simulink model "pi_choiceIface"  (R2018b)
settings: Solver=FixedStepDiscrete  StartTime=0.0  StopTime=10.0  RelTol=1e-3
undefined symbols (not defined in the file): boolAliasMember, boolMember, choiceAliasesMember, choiceBuiltInMember, choiceIdx, choiceOfFixedSizeSeqOfsMember, choiceOfVarSizeSeqOfsMember, enumAliasMember, enumMember, ia5StringFixedSizeAliasMember, ia5StringFixedSizeMember, ia5StringVarSizeAliasMember, ia5StringVarSizeMember, integerAliasMember, integerMember, octetStringFixedSizeAliasMember, octetStringFixedSizeMember, octetStringVarSizeAliasMember, octetStringVarSizeMember, realAliasMember, realMember, seqAliasesMember, seqBuiltInMember, seqOfFixedSizeSeqOfsMember, seqOfVarSizeSeqOfsMember
settings Model: Creator=matlab  LastModifiedBy=matlab
settings DataIOCC: SaveOutput=off  SignalLogging=off  SaveTime=off
settings OptimizationCC: DefaultParameterBehavior=Inlined  EnhancedBackFolding=on  PassReuseOutputArgsAs=Individual arguments  OptimizeBlockOrder=speed  DifferentSizesBufferReuse=on  OptimizationCustomize=off
settings DebuggingCC: ParameterTunabilityLossMsg=error
settings SFSimCC: MATLABDynamicMemAlloc=off
settings RTWCC: SystemTargetFile=ert.tlc  TemplateMakefile=ert_default_tmf  PostCodeGenCommand=packNGo(buildInfo);  GenerateReport=on  IncludeHyperlinkInReport=on  LaunchReport=on  GenerateTraceInfo=on  GenerateTraceReport=on  GenerateTraceReportSl=on  GenerateTraceReportSf=on  GenerateTraceReportEml=on
settings CodeAppCC: ForceParamTrailComments=on  IgnoreCustomStorageClasses=off  OperatorAnnotations=on  SimulinkDataObjDesc=on  SFDataObjDesc=on  InsertBlockDesc=on
settings ERTTargetCC: TargetLangStandard=C99 (ISO)  GenerateSampleERTMain=on  InlinedParameterPlacement=NonHierarchical  ERTCustomFileTemplate=example_file_process.tlc

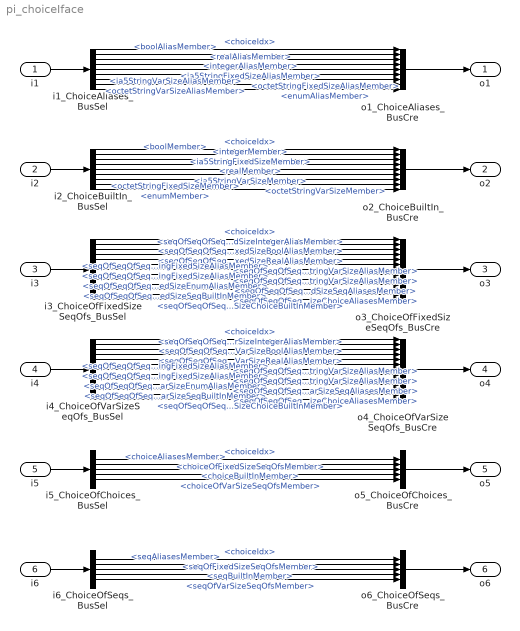
== system pi_choiceIface ==
  i1 : Inport  OutDataTypeStr=Bus: ChoiceAliases  BusOutputAsStruct=on
  i2 : Inport  Port=2  OutDataTypeStr=Bus: ChoiceBuiltIn  BusOutputAsStruct=on
  i3 : Inport  Port=3  OutDataTypeStr=Bus: ChoiceOfFixedSizeSeqOfs  BusOutputAsStruct=on
  i4 : Inport  Port=4  OutDataTypeStr=Bus: ChoiceOfVarSizeSeqOfs  BusOutputAsStruct=on
  i5 : Inport  Port=5  OutDataTypeStr=Bus: ChoiceOfChoices  BusOutputAsStruct=on
  i6 : Inport  Port=6  OutDataTypeStr=Bus: ChoiceOfSeqs  BusOutputAsStruct=on
  i1_ChoiceAliases_BusSel : BusSelector  OutputSignals=choiceIdx,boolAliasMember,integerAliasMember,realAliasMember,ia5StringFixedSizeAliasMember,ia5StringVarSizeAliasMember,octetStringFixedSizeAliasMember,octetStringVarSizeAliasMember,enumAliasMember
  i2_ChoiceBuiltIn_BusSel : BusSelector  OutputSignals=choiceIdx,boolMember,integerMember,realMember,ia5StringFixedSizeMember,ia5StringVarSizeMember,octetStringFixedSizeMember,octetStringVarSizeMember,enumMember
  i3_ChoiceOfFixedSizeSeqOfs_BusSel : BusSelector  OutputSignals=choiceIdx,seqOfSeqOfSeqOfFixedSizeBoolAliasMember,seqOfSeqOfSeqOfFixedSizeIntegerAliasMember,seqOfSeqOfSeqOfFixedSizeRealAliasMember,seqOfSeqOfSeqOfFixedSizeIA5StringFixedSizeAliasMember,seqOfSeqOfSeqOfFixedSizeIA5StringVarSizeAliasMember,seqOfSeqOfSeqOfFixedSizeOctetStringFixedSizeAliasMember,seqOfSeqOfSeqOfFixedSizeOctetStringVarSizeAliasMember,seqOfSeqOfSeqOfFixedSizeEnumAliasMember,seqOfSeqOfSeqOfFixedSizeSeqAliasesMember,seqOfSeqOfSeqOfFixedSizeSeqBuiltInMember,seqOfSeqOfSeqOfFixedSizeChoiceAliasesMember,seqOfSeqOfSeqOfFixedSizeChoiceBuiltInMember
  i4_ChoiceOfVarSizeSeqOfs_BusSel : BusSelector  OutputSignals=choiceIdx,seqOfSeqOfSeqOfVarSizeBoolAliasMember,seqOfSeqOfSeqOfVarSizeIntegerAliasMember,seqOfSeqOfSeqOfVarSizeRealAliasMember,seqOfSeqOfSeqOfVarSizeIA5StringFixedSizeAliasMember,seqOfSeqOfSeqOfVarSizeIA5StringVarSizeAliasMember,seqOfSeqOfSeqOfVarSizeOctetStringFixedSizeAliasMember,seqOfSeqOfSeqOfVarSizeOctetStringVarSizeAliasMember,seqOfSeqOfSeqOfVarSizeEnumAliasMember,seqOfSeqOfSeqOfVarSizeSeqAliasesMember,seqOfSeqOfSeqOfVarSizeSeqBuiltInMember,seqOfSeqOfSeqOfVarSizeChoiceAliasesMember,seqOfSeqOfSeqOfVarSizeChoiceBuiltInMember
  i5_ChoiceOfChoices_BusSel : BusSelector  OutputSignals=choiceIdx,choiceAliasesMember,choiceBuiltInMember,choiceOfFixedSizeSeqOfsMember,choiceOfVarSizeSeqOfsMember
  i6_ChoiceOfSeqs_BusSel : BusSelector  OutputSignals=choiceIdx,seqAliasesMember,seqBuiltInMember,seqOfFixedSizeSeqOfsMember,seqOfVarSizeSeqOfsMember
  o1_ChoiceAliases_BusCre : BusCreator  Inputs=choiceIdx,boolAliasMember,integerAliasMember,realAliasMember,ia5StringFixedSizeAliasMember,ia5StringVarSizeAliasMember,octetStringFixedSizeAliasMember,octetStringVarSizeAliasMember,enumAliasMember  OutDataTypeStr=Bus: ChoiceAliases  NonVirtualBus=on
  o2_ChoiceBuiltIn_BusCre : BusCreator  Inputs=choiceIdx,boolMember,integerMember,realMember,ia5StringFixedSizeMember,ia5StringVarSizeMember,octetStringFixedSizeMember,octetStringVarSizeMember,enumMember  OutDataTypeStr=Bus: ChoiceBuiltIn  NonVirtualBus=on
  o3_ChoiceOfFixedSizeSeqOfs_BusCre : BusCreator  Inputs=choiceIdx,seqOfSeqOfSeqOfFixedSizeBoolAliasMember,seqOfSeqOfSeqOfFixedSizeIntegerAliasMember,seqOfSeqOfSeqOfFixedSizeRealAliasMember,seqOfSeqOfSeqOfFixedSizeIA5StringFixedSizeAliasMember,seqOfSeqOfSeqOfFixedSizeIA5StringVarSizeAliasMember,seqOfSeqOfSeqOfFixedSizeOctetStringFixedSizeAliasMember,seqOfSeqOfSeqOfFixedSizeOctetStringVarSizeAliasMember,seqOfSeqOfSeqOfFixedSizeEnumAliasMember,seqOfSeqOfSeqOfFixedSizeSeqAliasesMember,seqOfSeqOfSeqOfFixedSizeSeqBuiltInMember,seqOfSeqOfSeqOfFixedSizeChoiceAliasesMember,seqOfSeqOfSeqOfFixedSizeChoiceBuiltInMember  OutDataTypeStr=Bus: ChoiceOfFixedSizeSeqOfs  NonVirtualBus=on
  o4_ChoiceOfVarSizeSeqOfs_BusCre : BusCreator  Inputs=choiceIdx,seqOfSeqOfSeqOfVarSizeBoolAliasMember,seqOfSeqOfSeqOfVarSizeIntegerAliasMember,seqOfSeqOfSeqOfVarSizeRealAliasMember,seqOfSeqOfSeqOfVarSizeIA5StringFixedSizeAliasMember,seqOfSeqOfSeqOfVarSizeIA5StringVarSizeAliasMember,seqOfSeqOfSeqOfVarSizeOctetStringFixedSizeAliasMember,seqOfSeqOfSeqOfVarSizeOctetStringVarSizeAliasMember,seqOfSeqOfSeqOfVarSizeEnumAliasMember,seqOfSeqOfSeqOfVarSizeSeqAliasesMember,seqOfSeqOfSeqOfVarSizeSeqBuiltInMember,seqOfSeqOfSeqOfVarSizeChoiceAliasesMember,seqOfSeqOfSeqOfVarSizeChoiceBuiltInMember  OutDataTypeStr=Bus: ChoiceOfVarSizeSeqOfs  NonVirtualBus=on
  o5_ChoiceOfChoices_BusCre : BusCreator  Inputs=choiceIdx,choiceAliasesMember,choiceBuiltInMember,choiceOfFixedSizeSeqOfsMember,choiceOfVarSizeSeqOfsMember  OutDataTypeStr=Bus: ChoiceOfChoices  NonVirtualBus=on
  o6_ChoiceOfSeqs_BusCre : BusCreator  Inputs=choiceIdx,seqAliasesMember,seqBuiltInMember,seqOfFixedSizeSeqOfsMember,seqOfVarSizeSeqOfsMember  OutDataTypeStr=Bus: ChoiceOfSeqs  NonVirtualBus=on
  o1 : Outport  OutDataTypeStr=Bus: ChoiceAliases  BusOutputAsStruct=on
  o2 : Outport  Port=2  OutDataTypeStr=Bus: ChoiceBuiltIn  BusOutputAsStruct=on
  o3 : Outport  Port=3  OutDataTypeStr=Bus: ChoiceOfFixedSizeSeqOfs  BusOutputAsStruct=on
  o4 : Outport  Port=4  OutDataTypeStr=Bus: ChoiceOfVarSizeSeqOfs  BusOutputAsStruct=on
  o5 : Outport  Port=5  OutDataTypeStr=Bus: ChoiceOfChoices  BusOutputAsStruct=on
  o6 : Outport  Port=6  OutDataTypeStr=Bus: ChoiceOfSeqs  BusOutputAsStruct=on
  wires:
  i1/1 -> i1_ChoiceAliases_BusSel/1
  i2/1 -> i2_ChoiceBuiltIn_BusSel/1
  i3/1 -> i3_ChoiceOfFixedSizeSeqOfs_BusSel/1
  i4/1 -> i4_ChoiceOfVarSizeSeqOfs_BusSel/1
  i5/1 -> i5_ChoiceOfChoices_BusSel/1
  i6/1 -> i6_ChoiceOfSeqs_BusSel/1
  o1_ChoiceAliases_BusCre/1 -> o1/1
  o2_ChoiceBuiltIn_BusCre/1 -> o2/1
  o3_ChoiceOfFixedSizeSeqOfs_BusCre/1 -> o3/1
  o4_ChoiceOfVarSizeSeqOfs_BusCre/1 -> o4/1
  o5_ChoiceOfChoices_BusCre/1 -> o5/1
  o6_ChoiceOfSeqs_BusCre/1 -> o6/1
  i1_ChoiceAliases_BusSel/1 -> o1_ChoiceAliases_BusCre/1  "<choiceIdx>"
  i1_ChoiceAliases_BusSel/2 -> o1_ChoiceAliases_BusCre/2  "<boolAliasMember>"
  i1_ChoiceAliases_BusSel/3 -> o1_ChoiceAliases_BusCre/3  "<integerAliasMember>"
  i1_ChoiceAliases_BusSel/4 -> o1_ChoiceAliases_BusCre/4  "<realAliasMember>"
  i1_ChoiceAliases_BusSel/5 -> o1_ChoiceAliases_BusCre/5  "<ia5StringFixedSizeAliasMember>"
  i1_ChoiceAliases_BusSel/6 -> o1_ChoiceAliases_BusCre/6  "<ia5StringVarSizeAliasMember>"
  i1_ChoiceAliases_BusSel/7 -> o1_ChoiceAliases_BusCre/7  "<octetStringFixedSizeAliasMember>"
  i1_ChoiceAliases_BusSel/8 -> o1_ChoiceAliases_BusCre/8  "<octetStringVarSizeAliasMember>"
  i1_ChoiceAliases_BusSel/9 -> o1_ChoiceAliases_BusCre/9  "<enumAliasMember>"
  i2_ChoiceBuiltIn_BusSel/1 -> o2_ChoiceBuiltIn_BusCre/1  "<choiceIdx>"
  i2_ChoiceBuiltIn_BusSel/2 -> o2_ChoiceBuiltIn_BusCre/2  "<boolMember>"
  i2_ChoiceBuiltIn_BusSel/3 -> o2_ChoiceBuiltIn_BusCre/3  "<integerMember>"
  i2_ChoiceBuiltIn_BusSel/4 -> o2_ChoiceBuiltIn_BusCre/4  "<realMember>"
  i2_ChoiceBuiltIn_BusSel/5 -> o2_ChoiceBuiltIn_BusCre/5  "<ia5StringFixedSizeMember>"
  i2_ChoiceBuiltIn_BusSel/6 -> o2_ChoiceBuiltIn_BusCre/6  "<ia5StringVarSizeMember>"
  i2_ChoiceBuiltIn_BusSel/7 -> o2_ChoiceBuiltIn_BusCre/7  "<octetStringFixedSizeMember>"
  i2_ChoiceBuiltIn_BusSel/8 -> o2_ChoiceBuiltIn_BusCre/8  "<octetStringVarSizeMember>"
  i2_ChoiceBuiltIn_BusSel/9 -> o2_ChoiceBuiltIn_BusCre/9  "<enumMember>"
  i3_ChoiceOfFixedSizeSeqOfs_BusSel/1 -> o3_ChoiceOfFixedSizeSeqOfs_BusCre/1  "<choiceIdx>"
  i3_ChoiceOfFixedSizeSeqOfs_BusSel/2 -> o3_ChoiceOfFixedSizeSeqOfs_BusCre/2  "<seqOfSeqOfSeqOfFixedSizeBoolAliasMember>"
  i3_ChoiceOfFixedSizeSeqOfs_BusSel/3 -> o3_ChoiceOfFixedSizeSeqOfs_BusCre/3  "<seqOfSeqOfSeqOfFixedSizeIntegerAliasMember>"
  i3_ChoiceOfFixedSizeSeqOfs_BusSel/4 -> o3_ChoiceOfFixedSizeSeqOfs_BusCre/4  "<seqOfSeqOfSeqOfFixedSizeRealAliasMember>"
  i3_ChoiceOfFixedSizeSeqOfs_BusSel/5 -> o3_ChoiceOfFixedSizeSeqOfs_BusCre/5  "<seqOfSeqOfSeqOfFixedSizeIA5StringFixedSizeAliasMember>"
  i3_ChoiceOfFixedSizeSeqOfs_BusSel/6 -> o3_ChoiceOfFixedSizeSeqOfs_BusCre/6  "<seqOfSeqOfSeqOfFixedSizeIA5StringVarSizeAliasMember>"
  i3_ChoiceOfFixedSizeSeqOfs_BusSel/7 -> o3_ChoiceOfFixedSizeSeqOfs_BusCre/7  "<seqOfSeqOfSeqOfFixedSizeOctetStringFixedSizeAliasMember>"
  i3_ChoiceOfFixedSizeSeqOfs_BusSel/8 -> o3_ChoiceOfFixedSizeSeqOfs_BusCre/8  "<seqOfSeqOfSeqOfFixedSizeOctetStringVarSizeAliasMember>"
  i3_ChoiceOfFixedSizeSeqOfs_BusSel/9 -> o3_ChoiceOfFixedSizeSeqOfs_BusCre/9  "<seqOfSeqOfSeqOfFixedSizeEnumAliasMember>"
  i3_ChoiceOfFixedSizeSeqOfs_BusSel/10 -> o3_ChoiceOfFixedSizeSeqOfs_BusCre/10  "<seqOfSeqOfSeqOfFixedSizeSeqAliasesMember>"
  i3_ChoiceOfFixedSizeSeqOfs_BusSel/11 -> o3_ChoiceOfFixedSizeSeqOfs_BusCre/11  "<seqOfSeqOfSeqOfFixedSizeSeqBuiltInMember>"
  i3_ChoiceOfFixedSizeSeqOfs_BusSel/12 -> o3_ChoiceOfFixedSizeSeqOfs_BusCre/12  "<seqOfSeqOfSeqOfFixedSizeChoiceAliasesMember>"
  i3_ChoiceOfFixedSizeSeqOfs_BusSel/13 -> o3_ChoiceOfFixedSizeSeqOfs_BusCre/13  "<seqOfSeqOfSeqOfFixedSizeChoiceBuiltInMember>"
  i4_ChoiceOfVarSizeSeqOfs_BusSel/1 -> o4_ChoiceOfVarSizeSeqOfs_BusCre/1  "<choiceIdx>"
  i4_ChoiceOfVarSizeSeqOfs_BusSel/2 -> o4_ChoiceOfVarSizeSeqOfs_BusCre/2  "<seqOfSeqOfSeqOfVarSizeBoolAliasMember>"
  i4_ChoiceOfVarSizeSeqOfs_BusSel/3 -> o4_ChoiceOfVarSizeSeqOfs_BusCre/3  "<seqOfSeqOfSeqOfVarSizeIntegerAliasMember>"
  i4_ChoiceOfVarSizeSeqOfs_BusSel/4 -> o4_ChoiceOfVarSizeSeqOfs_BusCre/4  "<seqOfSeqOfSeqOfVarSizeRealAliasMember>"
  i4_ChoiceOfVarSizeSeqOfs_BusSel/5 -> o4_ChoiceOfVarSizeSeqOfs_BusCre/5  "<seqOfSeqOfSeqOfVarSizeIA5StringFixedSizeAliasMember>"
  i4_ChoiceOfVarSizeSeqOfs_BusSel/6 -> o4_ChoiceOfVarSizeSeqOfs_BusCre/6  "<seqOfSeqOfSeqOfVarSizeIA5StringVarSizeAliasMember>"
  i4_ChoiceOfVarSizeSeqOfs_BusSel/7 -> o4_ChoiceOfVarSizeSeqOfs_BusCre/7  "<seqOfSeqOfSeqOfVarSizeOctetStringFixedSizeAliasMember>"
  i4_ChoiceOfVarSizeSeqOfs_BusSel/8 -> o4_ChoiceOfVarSizeSeqOfs_BusCre/8  "<seqOfSeqOfSeqOfVarSizeOctetStringVarSizeAliasMember>"
  i4_ChoiceOfVarSizeSeqOfs_BusSel/9 -> o4_ChoiceOfVarSizeSeqOfs_BusCre/9  "<seqOfSeqOfSeqOfVarSizeEnumAliasMember>"
  i4_ChoiceOfVarSizeSeqOfs_BusSel/10 -> o4_ChoiceOfVarSizeSeqOfs_BusCre/10  "<seqOfSeqOfSeqOfVarSizeSeqAliasesMember>"
  i4_ChoiceOfVarSizeSeqOfs_BusSel/11 -> o4_ChoiceOfVarSizeSeqOfs_BusCre/11  "<seqOfSeqOfSeqOfVarSizeSeqBuiltInMember>"
  i4_ChoiceOfVarSizeSeqOfs_BusSel/12 -> o4_ChoiceOfVarSizeSeqOfs_BusCre/12  "<seqOfSeqOfSeqOfVarSizeChoiceAliasesMember>"
  i4_ChoiceOfVarSizeSeqOfs_BusSel/13 -> o4_ChoiceOfVarSizeSeqOfs_BusCre/13  "<seqOfSeqOfSeqOfVarSizeChoiceBuiltInMember>"
  i5_ChoiceOfChoices_BusSel/1 -> o5_ChoiceOfChoices_BusCre/1  "<choiceIdx>"
  i5_ChoiceOfChoices_BusSel/2 -> o5_ChoiceOfChoices_BusCre/2  "<choiceAliasesMember>"
  i5_ChoiceOfChoices_BusSel/3 -> o5_ChoiceOfChoices_BusCre/3  "<choiceBuiltInMember>"
  i5_ChoiceOfChoices_BusSel/4 -> o5_ChoiceOfChoices_BusCre/4  "<choiceOfFixedSizeSeqOfsMember>"
  i5_ChoiceOfChoices_BusSel/5 -> o5_ChoiceOfChoices_BusCre/5  "<choiceOfVarSizeSeqOfsMember>"
  i6_ChoiceOfSeqs_BusSel/1 -> o6_ChoiceOfSeqs_BusCre/1  "<choiceIdx>"
  i6_ChoiceOfSeqs_BusSel/2 -> o6_ChoiceOfSeqs_BusCre/2  "<seqAliasesMember>"
  i6_ChoiceOfSeqs_BusSel/3 -> o6_ChoiceOfSeqs_BusCre/3  "<seqBuiltInMember>"
  i6_ChoiceOfSeqs_BusSel/4 -> o6_ChoiceOfSeqs_BusCre/4  "<seqOfFixedSizeSeqOfsMember>"
  i6_ChoiceOfSeqs_BusSel/5 -> o6_ChoiceOfSeqs_BusCre/5  "<seqOfVarSizeSeqOfsMember>"
